simulink library "Enrg_conv_El_to_Mec_Bosch"  (R2016a)
settings: Solver=ode1  StartTime=0.0  StopTime=Inf  FixedStep=0.001  RelTol=1e-3
undefined symbols (not defined in the file): drvEmot_RefTqeMOT, FirstDrivenAxle_FirstDrivenAxleNoOfEmot, FMIKit, SecondDrivenAxle_SecondDrivenAxleNoOfEmot
libraries: Enrg_conv_El_to_Mec_Bosch x13, Electrical_converter x8
(part 4 of 5)

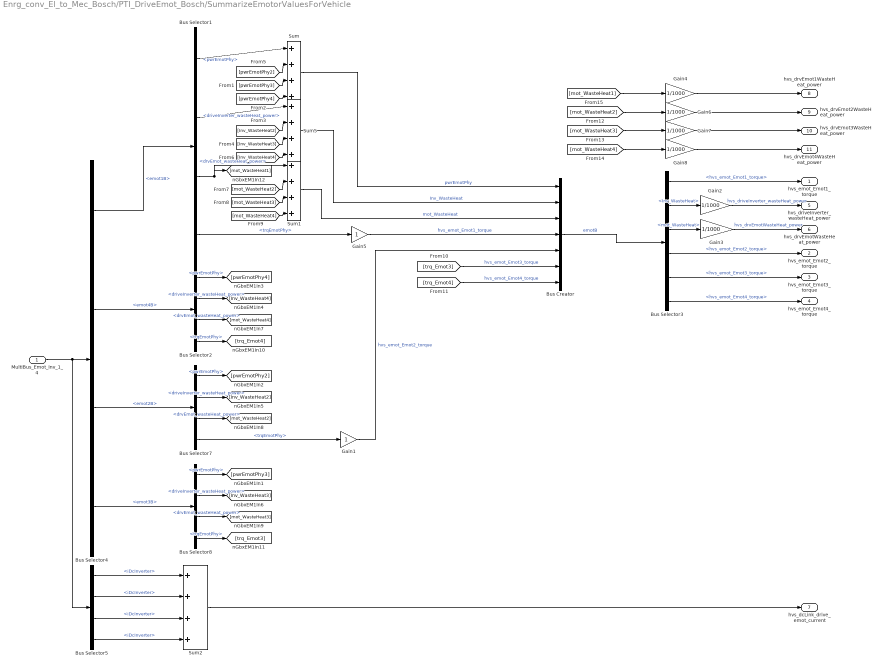
== system Enrg_conv_El_to_Mec_Bosch/PTI_DriveEmot_Bosch/SummarizeEmotorValuesForVehicle ==
  MultiBus_Emot_Inv_1_4 : Inport
  Bus Creator : BusCreator  Inputs=7
  Bus Selector{1..2,7..8} (4 alike) : BusSelector  OutputSignals=pwrEmotPhy,driveInverter_wasteHeat_power,drvEmot_wasteHeat_power,trqEmotPhy
  Bus Selector3 : BusSelector  OutputSignals=hvs_emot_Emot1_torque,Inv_WasteHeat,mot_WasteHeat,hvs_emot_Emot2_torque,hvs_emot_Emot3_torque,hvs_emot_Emot4_torque
  Bus Selector4 : BusSelector  OutputSignals=emot1_4B.emot1B,emot1_4B.emot4B,emot2_3B.emot2B,emot2_3B.emot3B
  Bus Selector5 : BusSelector  OutputSignals=emot1_4B.emot1B.iDcInverter,emot1_4B.emot4B.iDcInverter,emot2_3B.emot2B.iDcInverter,emot2_3B.emot3B.iDcInverter
  Gain1 : Gain
  Gain{2..4,6..8} (6 alike) : Gain  Gain=1/1000
  Gain5 : Gain
  Sum : Sum  Inputs=|++++
  Sum1 : Sum  Inputs=|++++
  Sum2 : Sum  Inputs=++++
  Sum5 : Sum  Inputs=|++++
  hvs_emot_Emot1_torque : Outport
  hvs_emot_Emot2_torque : Outport  Port=2
  hvs_emot_Emot3_torque : Outport  Port=3
  hvs_emot_Emot4_torque : Outport  Port=4
  hvs_driveInverter_wasteHeat_power : Outport  Port=5
  hvs_drvEmotWasteHeat_power : Outport  Port=6
  hvs_dcLink_drive_emot_current : Outport  Port=7
  hvs_drvEmot1WasteHeat_power : Outport  Port=8
  hvs_drvEmot2WasteHeat_power : Outport  Port=9
  hvs_drvEmot3WasteHeat_power : Outport  Port=10
  hvs_drvEmot4WasteHeat_power : Outport  Port=11
  wires:
  Gain5/1 -> Bus Creator/4  "hvs_emot_Emot1_torque"
  Sum1/1 -> Bus Creator/3  "mot_WasteHeat"
  Sum5/1 -> Bus Creator/2  "Inv_WasteHeat"
  Sum/1 -> Bus Creator/1  "pwrEmotPhy"
  Bus Selector1/4 -> Gain5/1  "<trqEmotPhy>"
  Bus Selector2/3 -> [mot_WasteHeat4]  "<drvEmot_wasteHeat_power>"
  Bus Selector1/3 -> [mot_WasteHeat1], Sum1/1  "<drvEmot_wasteHeat_power>"
  Bus Selector2/2 -> [Inv_WasteHeat4]  "<driveInverter_wasteHeat_power>"
  Bus Selector1/2 -> Sum5/1  "<driveInverter_wasteHeat_power>"
  Bus Selector1/1 -> Sum/1  "<pwrEmotPhy>"
  Bus Selector4/2 -> Bus Selector2/1  "<emot4B>"
  Bus Selector4/1 -> Bus Selector1/1  "<emot1B>"
  MultiBus_Emot_Inv_1_4/1 -> Bus Selector5/1, Bus Selector4/1
  Bus Creator/1 -> Bus Selector3/1  "emotB"
  Sum2/1 -> hvs_dcLink_drive_emot_current/1
  Bus Selector3/2 -> Gain2/1  "<Inv_WasteHeat>"
  Gain2/1 -> hvs_driveInverter_wasteHeat_power/1  "hvs_driveInverter_wasteHeat_power"
  Bus Selector3/3 -> Gain3/1  "<mot_WasteHeat>"
  Gain3/1 -> hvs_drvEmotWasteHeat_power/1  "hvs_drvEmotWasteHeat_power"
  Bus Selector4/4 -> Bus Selector8/1  "<emot3B>"
  Bus Selector4/3 -> Bus Selector7/1  "<emot2B>"
  Bus Selector7/1 -> [pwrEmotPhy2]  "<pwrEmotPhy>"
  Bus Selector8/1 -> [pwrEmotPhy3]  "<pwrEmotPhy>"
  Bus Selector2/1 -> [pwrEmotPhy4]  "<pwrEmotPhy>"
  [pwrEmotPhy2] -> Sum/2
  [pwrEmotPhy3] -> Sum/3
  [pwrEmotPhy4] -> Sum/4
  [Inv_WasteHeat2] -> Sum5/2
  [Inv_WasteHeat3] -> Sum5/3
  [Inv_WasteHeat4] -> Sum5/4
  Bus Selector7/2 -> [Inv_WasteHeat2]  "<driveInverter_wasteHeat_power>"
  Bus Selector8/2 -> [Inv_WasteHeat3]  "<driveInverter_wasteHeat_power>"
  Bus Selector7/3 -> [mot_WasteHeat2]  "<drvEmot_wasteHeat_power>"
  Bus Selector8/3 -> [mot_WasteHeat3]  "<drvEmot_wasteHeat_power>"
  [mot_WasteHeat2] -> Sum1/2
  [mot_WasteHeat3] -> Sum1/3
  [mot_WasteHeat4] -> Sum1/4
  Bus Selector7/4 -> Gain1/1  "<trqEmotPhy>"
  Bus Selector8/4 -> [trq_Emot3]  "<trqEmotPhy>"
  Gain1/1 -> Bus Creator/5  "hvs_emot_Emot2_torque"
  Bus Selector2/4 -> [trq_Emot4]  "<trqEmotPhy>"
  [trq_Emot3] -> Bus Creator/6  "hvs_emot_Emot3_torque"
  [trq_Emot4] -> Bus Creator/7  "hvs_emot_Emot4_torque"
  Bus Selector3/1 -> hvs_emot_Emot1_torque/1  "<hvs_emot_Emot1_torque>"
  Bus Selector3/4 -> hvs_emot_Emot2_torque/1  "<hvs_emot_Emot2_torque>"
  Bus Selector3/5 -> hvs_emot_Emot3_torque/1  "<hvs_emot_Emot3_torque>"
  Bus Selector3/6 -> hvs_emot_Emot4_torque/1  "<hvs_emot_Emot4_torque>"
  [mot_WasteHeat1] -> Gain4/1
  [mot_WasteHeat2] -> Gain6/1
  [mot_WasteHeat3] -> Gain7/1
  [mot_WasteHeat4] -> Gain8/1
  Gain4/1 -> hvs_drvEmot1WasteHeat_power/1
  Gain6/1 -> hvs_drvEmot2WasteHeat_power/1
  Gain7/1 -> hvs_drvEmot3WasteHeat_power/1
  Gain8/1 -> hvs_drvEmot4WasteHeat_power/1
  Bus Selector5/1 -> Sum2/1  "<iDcInverter>"
  Bus Selector5/3 -> Sum2/3  "<iDcInverter>"
  Bus Selector5/4 -> Sum2/4  "<iDcInverter>"
  Bus Selector5/2 -> Sum2/2  "<iDcInverter>"

== system Enrg_conv_El_to_Mec_Bosch/PTI_DriveEmot_Bosch_10ms/AWR1_4 ==
  EMD1_CMD_Commamd : Inport
  EMD1_CMD_MotorControlMode : Inport  Port=2
  EMD1_CMD_SpeedRefLim : Inport  Port=3
  EMD1_CMD_TorqueRefLim : Inport  Port=4
  HVFreigabeHW_SiRelay_D : Inport  Port=5
  vltZkBmsPhy : Inport  Port=6
  trqEmot1Phy : Inport  Port=7
  trqEmot4Phy : Inport  Port=8
  pwEmot1Phy : Inport  Port=9
  pwEmot4Phy : Inport  Port=10
  trqEmot1Max : Inport  Port=11
  trqEmot4Max : Inport  Port=12
  hvs_emot_Emot1_angVel : Inport  Port=13
  EMD4_CMD_Commamd : Inport  Port=14
  EMD4_CMD_MotorControlMode : Inport  Port=15
  EMD4_CMD_SpeedRefLim : Inport  Port=16
  EMD4_CMD_TorqueRefLim : Inport  Port=17
  HVFreigabeHW4_SiRelay_D : Inport  Port=18
  EDCU_Dig_SafetyCutOffDG1 : Inport  Port=19
  Emot1_Selection : Inport  Port=20
  Emot4_Selection : Inport  Port=21
  hvs_emot_Emot4_angVel : Inport  Port=22
  Bus Creator3 : BusCreator  Inputs=11
  Bus Creator4 : BusCreator  Inputs=2
  Bus Creator5 : BusCreator  Inputs=11
  Gain : Gain
  Gain1 : Gain
  Switch1 : Switch  Threshold=0.5
  Switch2 : Switch  Threshold=0.5
  ZeroWhenNotReady1 : Subsystem  TreatAsAtomicUnit=on
  ZeroWhenNotReady2 : Subsystem  TreatAsAtomicUnit=on
  awr1 : Electrical_converter/awr  SystemSampleTime=-1
  awr4 : Electrical_converter/awr  SystemSampleTime=-1
  awr1_4B : Outport
  wires:
  Emot1_Selection/1 -> awr1/Enable
  Emot4_Selection/1 -> awr4/Enable
  [EDCU_Dig_SafetyCutOffDG1] -> awr4/11
  EDCU_Dig_SafetyCutOffDG1/1 -> awr1/11, [EDCU_Dig_SafetyCutOffDG1]
  [vltZkBmsPhy] -> awr4/6
  EMD1_CMD_Commamd/1 -> awr1/1
  Bus Creator5/1 -> Switch2/1
  awr1/12 -> Switch2/2
  awr1/2 -> Bus Creator5/2
  awr1/3 -> Bus Creator5/3
  awr1/1 -> Gain/1
  awr1/4 -> Bus Creator5/4
  awr1/5 -> Bus Creator5/5
  awr1/8 -> Bus Creator5/8
  awr1/11 -> Bus Creator5/11
  awr1/10 -> Bus Creator5/10
  awr1/6 -> Bus Creator5/6
  awr1/7 -> Bus Creator5/7
  awr1/9 -> Bus Creator5/9
  awr4/12 -> Switch1/2
  Switch2/1 -> Bus Creator4/1  "awr1B"
  ZeroWhenNotReady1/1(Out1) -> Switch2/3
  awr4/4 -> Bus Creator3/4
  awr4/1 -> Gain1/1
  awr4/6 -> Bus Creator3/6
  awr4/7 -> Bus Creator3/7
  awr4/8 -> Bus Creator3/8
  awr4/9 -> Bus Creator3/9
  awr4/5 -> Bus Creator3/5
  awr4/11 -> Bus Creator3/11
  awr4/10 -> Bus Creator3/10
  awr4/3 -> Bus Creator3/3
  awr4/2 -> Bus Creator3/2
  Switch1/1 -> Bus Creator4/2  "awr4B"
  ZeroWhenNotReady2/1(Out1) -> Switch1/3
  Bus Creator3/1 -> Switch1/1  "awr4B"
  trqEmot1Max/1 -> awr1/9
  pwEmot1Phy/1 -> awr1/8
  trqEmot1Phy/1 -> awr1/7
  trqEmot4Max/1 -> awr4/9
  pwEmot4Phy/1 -> awr4/8
  trqEmot4Phy/1 -> awr4/7
  Bus Creator4/1 -> awr1_4B/1  "awr1_4B"
  EMD4_CMD_TorqueRefLim/1 -> awr4/4
  EMD4_CMD_Commamd/1 -> awr4/1
  EMD4_CMD_SpeedRefLim/1 -> awr4/3
  HVFreigabeHW4_SiRelay_D/1 -> awr4/5
  HVFreigabeHW_SiRelay_D/1 -> awr1/5
  EMD1_CMD_TorqueRefLim/1 -> awr1/4
  EMD1_CMD_SpeedRefLim/1 -> awr1/3
  Gain/1 -> Bus Creator5/1  "EMD1_ACT_DcLinkVoltage"
  Gain1/1 -> Bus Creator3/1  "EMD4_ACT_DcLinkVoltage"
  hvs_emot_Emot4_angVel/1 -> awr4/10
  EMD4_CMD_MotorControlMode/1 -> awr4/2
  EMD1_CMD_MotorControlMode/1 -> awr1/2
  vltZkBmsPhy/1 -> awr1/6, [vltZkBmsPhy]
  hvs_emot_Emot1_angVel/1 -> awr1/10

== system Enrg_conv_El_to_Mec_Bosch/PTI_DriveEmot_Bosch_10ms/AWR2_3 ==
  EMD2_CMD_Commamd : Inport
  EMD2_CMD_MotorControlMode : Inport  Port=2
  EMD2_CMD_SpeedRefLim : Inport  Port=3
  EMD2_CMD_TorqueRefLim : Inport  Port=4
  HVFreigabeHW2_SiRelay_D : Inport  Port=5
  vltZkBmsPhy : Inport  Port=6
  trqEmot2Phy : Inport  Port=7
  trqEmot3Phy : Inport  Port=8
  pwEmot2Phy : Inport  Port=9
  pwEmot3Phy : Inport  Port=10
  trqEmot2Max : Inport  Port=11
  trqEmot3Max : Inport  Port=12
  hvs_emot_Emot2_angVel : Inport  Port=13
  EMD3_CMD_Commamd : Inport  Port=14
  EMD3_CMD_MotorControlMode : Inport  Port=15
  EMD3_CMD_SpeedRefLim : Inport  Port=16
  EMD3_CMD_TorqueRefLim : Inport  Port=17
  HVFreigabeHW3_SiRelay_D : Inport  Port=18
  EDCU_Dig_SafetyCutOffDG1 : Inport  Port=19
  Emot2_Selection : Inport  Port=20
  Emot3_Selection : Inport  Port=21
  hvs_emot_Emot3_angVel : Inport  Port=22
  Bus Creator3 : BusCreator  Inputs=11
  Bus Creator4 : BusCreator  Inputs=2
  Bus Creator5 : BusCreator  Inputs=11
  Gain : Gain
  Gain1 : Gain
  Switch1 : Switch  Threshold=0.5
  Switch2 : Switch  Threshold=0.5
  ZeroWhenNotReady1 : Subsystem  TreatAsAtomicUnit=on
  ZeroWhenNotReady2 : Subsystem  TreatAsAtomicUnit=on
  awr2 : Electrical_converter/awr  SystemSampleTime=-1
  awr3 : Electrical_converter/awr  SystemSampleTime=-1
  awr2_3B : Outport
  wires:
  Emot3_Selection/1 -> awr3/Enable
  Emot2_Selection/1 -> awr2/Enable
  [EDCU_Dig_SafetyCutOffDG1] -> awr3/11
  EDCU_Dig_SafetyCutOffDG1/1 -> awr2/11, [EDCU_Dig_SafetyCutOffDG1]
  hvs_emot_Emot2_angVel/1 -> awr2/10
  vltZkBmsPhy/1 -> [vltZkBmsPhy], awr2/6
  EMD2_CMD_MotorControlMode/1 -> awr2/2
  EMD3_CMD_MotorControlMode/1 -> awr3/2
  hvs_emot_Emot3_angVel/1 -> awr3/10
  Gain1/1 -> Bus Creator3/1  "EMD3_ACT_DcLinkVoltage"
  Gain/1 -> Bus Creator5/1  "EMD2_ACT_DcLinkVoltage"
  EMD2_CMD_SpeedRefLim/1 -> awr2/3
  EMD2_CMD_TorqueRefLim/1 -> awr2/4
  HVFreigabeHW2_SiRelay_D/1 -> awr2/5
  HVFreigabeHW3_SiRelay_D/1 -> awr3/5
  EMD3_CMD_SpeedRefLim/1 -> awr3/3
  EMD3_CMD_Commamd/1 -> awr3/1
  EMD3_CMD_TorqueRefLim/1 -> awr3/4
  Bus Creator4/1 -> awr2_3B/1  "awr2_3B"
  trqEmot3Phy/1 -> awr3/7
  pwEmot3Phy/1 -> awr3/8
  trqEmot3Max/1 -> awr3/9
  trqEmot2Phy/1 -> awr2/7
  pwEmot2Phy/1 -> awr2/8
  trqEmot2Max/1 -> awr2/9
  Bus Creator3/1 -> Switch1/1  "awr3B"
  ZeroWhenNotReady2/1(Out1) -> Switch1/3
  Switch1/1 -> Bus Creator4/2  "awr3B"
  awr3/2 -> Bus Creator3/2
  awr3/3 -> Bus Creator3/3
  awr3/10 -> Bus Creator3/10
  awr3/11 -> Bus Creator3/11
  awr3/5 -> Bus Creator3/5
  awr3/9 -> Bus Creator3/9
  awr3/8 -> Bus Creator3/8
  awr3/7 -> Bus Creator3/7
  awr3/6 -> Bus Creator3/6
  awr3/1 -> Gain1/1
  awr3/4 -> Bus Creator3/4
  ZeroWhenNotReady1/1(Out1) -> Switch2/3
  Switch2/1 -> Bus Creator4/1  "awr2B"
  awr3/12 -> Switch1/2
  awr2/9 -> Bus Creator5/9
  awr2/7 -> Bus Creator5/7
  awr2/6 -> Bus Creator5/6
  awr2/10 -> Bus Creator5/10
  awr2/11 -> Bus Creator5/11
  awr2/8 -> Bus Creator5/8
  awr2/5 -> Bus Creator5/5
  awr2/4 -> Bus Creator5/4
  awr2/1 -> Gain/1
  awr2/3 -> Bus Creator5/3
  awr2/2 -> Bus Creator5/2
  awr2/12 -> Switch2/2
  Bus Creator5/1 -> Switch2/1
  EMD2_CMD_Commamd/1 -> awr2/1
  [vltZkBmsPhy] -> awr3/6

== system Enrg_conv_El_to_Mec_Bosch/PTI_DriveEmot_Bosch_10ms/EMD1_CMD_Command ==
  EMD1_CMD_ClearErrors : Inport
  EMD1_CMD_MotorControlMode : Inport  Port=2
  Compare To Constant : Subsystem  mask(Compare To Constant){relop===, const=1, OutDataTypeStr=boolean, ZeroCross=on}
      mask prompts: relop "Simulink:masks:Operator_MP"; const "Simulink:masks:ConstantValue_MP"; OutDataTypeStr "Simulink:masks:OutputDataType_MP"; ZeroCross "Simulink:masks:EnableZerocrossingDetection_MP"
      mask help: Simulink:masks:CompareToConstant_MD
      mask init: same as Enrg_conv_El_to_Mec_Bosch/PTI_DriveEmot_Bosch/EMD1_CMD_Command/Compare To Constant
      mask TypeOptions relop: == | ~= | < | <= | >= | >
      mask TypeOptions OutDataTypeStr: Simulink:masks:uint8 | Simulink:masks:boolean
      mask Callback ZeroCross: sl('zeroCrossEnable', gcbh);
      mask Display: disp(str)
  Compare To Constant1 : Subsystem  mask(Compare To Constant){relop===, const=1, OutDataTypeStr=boolean, ZeroCross=on}
      mask prompts: relop "Simulink:masks:Operator_MP"; const "Simulink:masks:ConstantValue_MP"; OutDataTypeStr "Simulink:masks:OutputDataType_MP"; ZeroCross "Simulink:masks:EnableZerocrossingDetection_MP"
      mask help: Simulink:masks:CompareToConstant_MD
      mask init: same as Enrg_conv_El_to_Mec_Bosch/PTI_DriveEmot_Bosch/EMD1_CMD_Command/Compare To Constant
      mask TypeOptions relop: == | ~= | < | <= | >= | >
      mask TypeOptions OutDataTypeStr: Simulink:masks:uint8 | Simulink:masks:boolean
      mask Callback ZeroCross: sl('zeroCrossEnable', gcbh);
      mask Display: disp(str)
  Constant : Constant  Value=4
  Constant3 : Constant
  Constant4 : Constant  Value=0
  Switch : Switch  Threshold=0.5
  Switch1 : Switch  Threshold=0.5
  Out_EMD1_CMD_Command : Outport
  wires:
  EMD1_CMD_MotorControlMode/1 -> Compare To Constant/1(u)
  EMD1_CMD_ClearErrors/1 -> Compare To Constant1/1(u)
  Compare To Constant1/1(y) -> Switch/2
  Switch1/1 -> Switch/3
  Constant/1 -> Switch/1
  Constant3/1 -> Switch1/1
  Constant4/1 -> Switch1/3
  Switch/1 -> Out_EMD1_CMD_Command/1
  Compare To Constant/1(y) -> Switch1/2

== system Enrg_conv_El_to_Mec_Bosch/PTI_DriveEmot_Bosch_10ms/EMD1_CMD_Command1 ==
  EMD1_CMD_ClearErrors : Inport
  EMD1_CMD_MotorControlMode : Inport  Port=2
  Compare To Constant : Subsystem  mask(Compare To Constant){relop===, const=1, OutDataTypeStr=boolean, ZeroCross=on}
      mask prompts: relop "Simulink:masks:Operator_MP"; const "Simulink:masks:ConstantValue_MP"; OutDataTypeStr "Simulink:masks:OutputDataType_MP"; ZeroCross "Simulink:masks:EnableZerocrossingDetection_MP"
      mask help: Simulink:masks:CompareToConstant_MD
      mask init: same as Enrg_conv_El_to_Mec_Bosch/PTI_DriveEmot_Bosch/EMD1_CMD_Command/Compare To Constant
      mask TypeOptions relop: == | ~= | < | <= | >= | >
      mask TypeOptions OutDataTypeStr: Simulink:masks:uint8 | Simulink:masks:boolean
      mask Callback ZeroCross: sl('zeroCrossEnable', gcbh);
      mask Display: disp(str)
  Compare To Constant1 : Subsystem  mask(Compare To Constant){relop===, const=1, OutDataTypeStr=boolean, ZeroCross=on}
      mask prompts: relop "Simulink:masks:Operator_MP"; const "Simulink:masks:ConstantValue_MP"; OutDataTypeStr "Simulink:masks:OutputDataType_MP"; ZeroCross "Simulink:masks:EnableZerocrossingDetection_MP"
      mask help: Simulink:masks:CompareToConstant_MD
      mask init: same as Enrg_conv_El_to_Mec_Bosch/PTI_DriveEmot_Bosch/EMD1_CMD_Command/Compare To Constant
      mask TypeOptions relop: == | ~= | < | <= | >= | >
      mask TypeOptions OutDataTypeStr: Simulink:masks:uint8 | Simulink:masks:boolean
      mask Callback ZeroCross: sl('zeroCrossEnable', gcbh);
      mask Display: disp(str)
  Constant : Constant  Value=4
  Constant3 : Constant
  Constant4 : Constant  Value=0
  Switch : Switch  Threshold=0.5
  Switch1 : Switch  Threshold=0.5
  Out_EMD1_CMD_Command : Outport
  wires:
  EMD1_CMD_MotorControlMode/1 -> Compare To Constant/1(u)
  EMD1_CMD_ClearErrors/1 -> Compare To Constant1/1(u)
  Compare To Constant1/1(y) -> Switch/2
  Switch1/1 -> Switch/3
  Constant/1 -> Switch/1
  Constant3/1 -> Switch1/1
  Constant4/1 -> Switch1/3
  Switch/1 -> Out_EMD1_CMD_Command/1
  Compare To Constant/1(y) -> Switch1/2

== system Enrg_conv_El_to_Mec_Bosch/PTI_DriveEmot_Bosch_10ms/EMD1_CMD_Command2 ==
  EMD1_CMD_ClearErrors : Inport
  EMD1_CMD_MotorControlMode : Inport  Port=2
  Compare To Constant : Subsystem  mask(Compare To Constant){relop===, const=1, OutDataTypeStr=boolean, ZeroCross=on}
      mask prompts: relop "Simulink:masks:Operator_MP"; const "Simulink:masks:ConstantValue_MP"; OutDataTypeStr "Simulink:masks:OutputDataType_MP"; ZeroCross "Simulink:masks:EnableZerocrossingDetection_MP"
      mask help: Simulink:masks:CompareToConstant_MD
      mask init: same as Enrg_conv_El_to_Mec_Bosch/PTI_DriveEmot_Bosch/EMD1_CMD_Command/Compare To Constant
      mask TypeOptions relop: == | ~= | < | <= | >= | >
      mask TypeOptions OutDataTypeStr: Simulink:masks:uint8 | Simulink:masks:boolean
      mask Callback ZeroCross: sl('zeroCrossEnable', gcbh);
      mask Display: disp(str)
  Compare To Constant1 : Subsystem  mask(Compare To Constant){relop===, const=1, OutDataTypeStr=boolean, ZeroCross=on}
      mask prompts: relop "Simulink:masks:Operator_MP"; const "Simulink:masks:ConstantValue_MP"; OutDataTypeStr "Simulink:masks:OutputDataType_MP"; ZeroCross "Simulink:masks:EnableZerocrossingDetection_MP"
      mask help: Simulink:masks:CompareToConstant_MD
      mask init: same as Enrg_conv_El_to_Mec_Bosch/PTI_DriveEmot_Bosch/EMD1_CMD_Command/Compare To Constant
      mask TypeOptions relop: == | ~= | < | <= | >= | >
      mask TypeOptions OutDataTypeStr: Simulink:masks:uint8 | Simulink:masks:boolean
      mask Callback ZeroCross: sl('zeroCrossEnable', gcbh);
      mask Display: disp(str)
  Constant : Constant  Value=4
  Constant3 : Constant
  Constant4 : Constant  Value=0
  Switch : Switch  Threshold=0.5
  Switch1 : Switch  Threshold=0.5
  Out_EMD1_CMD_Command : Outport
  wires:
  EMD1_CMD_MotorControlMode/1 -> Compare To Constant/1(u)
  EMD1_CMD_ClearErrors/1 -> Compare To Constant1/1(u)
  Compare To Constant1/1(y) -> Switch/2
  Switch1/1 -> Switch/3
  Constant/1 -> Switch/1
  Constant3/1 -> Switch1/1
  Constant4/1 -> Switch1/3
  Switch/1 -> Out_EMD1_CMD_Command/1
  Compare To Constant/1(y) -> Switch1/2

== system Enrg_conv_El_to_Mec_Bosch/PTI_DriveEmot_Bosch_10ms/EMD1_CMD_Command3 ==
  EMD1_CMD_ClearErrors : Inport
  EMD1_CMD_MotorControlMode : Inport  Port=2
  Compare To Constant : Subsystem  mask(Compare To Constant){relop===, const=1, OutDataTypeStr=boolean, ZeroCross=on}
      mask prompts: relop "Simulink:masks:Operator_MP"; const "Simulink:masks:ConstantValue_MP"; OutDataTypeStr "Simulink:masks:OutputDataType_MP"; ZeroCross "Simulink:masks:EnableZerocrossingDetection_MP"
      mask help: Simulink:masks:CompareToConstant_MD
      mask init: same as Enrg_conv_El_to_Mec_Bosch/PTI_DriveEmot_Bosch/EMD1_CMD_Command/Compare To Constant
      mask TypeOptions relop: == | ~= | < | <= | >= | >
      mask TypeOptions OutDataTypeStr: Simulink:masks:uint8 | Simulink:masks:boolean
      mask Callback ZeroCross: sl('zeroCrossEnable', gcbh);
      mask Display: disp(str)
  Compare To Constant1 : Subsystem  mask(Compare To Constant){relop===, const=1, OutDataTypeStr=boolean, ZeroCross=on}
      mask prompts: relop "Simulink:masks:Operator_MP"; const "Simulink:masks:ConstantValue_MP"; OutDataTypeStr "Simulink:masks:OutputDataType_MP"; ZeroCross "Simulink:masks:EnableZerocrossingDetection_MP"
      mask help: Simulink:masks:CompareToConstant_MD
      mask init: same as Enrg_conv_El_to_Mec_Bosch/PTI_DriveEmot_Bosch/EMD1_CMD_Command/Compare To Constant
      mask TypeOptions relop: == | ~= | < | <= | >= | >
      mask TypeOptions OutDataTypeStr: Simulink:masks:uint8 | Simulink:masks:boolean
      mask Callback ZeroCross: sl('zeroCrossEnable', gcbh);
      mask Display: disp(str)
  Constant : Constant  Value=4
  Constant3 : Constant
  Constant4 : Constant  Value=0
  Switch : Switch  Threshold=0.5
  Switch1 : Switch  Threshold=0.5
  Out_EMD1_CMD_Command : Outport
  wires:
  EMD1_CMD_MotorControlMode/1 -> Compare To Constant/1(u)
  EMD1_CMD_ClearErrors/1 -> Compare To Constant1/1(u)
  Compare To Constant1/1(y) -> Switch/2
  Switch1/1 -> Switch/3
  Constant/1 -> Switch/1
  Constant3/1 -> Switch1/1
  Constant4/1 -> Switch1/3
  Switch/1 -> Out_EMD1_CMD_Command/1
  Compare To Constant/1(y) -> Switch1/2

== system Enrg_conv_El_to_Mec_Bosch/PTI_DriveEmot_Bosch_10ms/Emot1_4 ==
  emot_Emot1_angVel : Inport
  voltBatHV1 : Inport  Port=2
  trqEmotDesPhy1 : Inport  Port=3
  voltBatHV4 : Inport  Port=4
  trqEmotDesPhy4 : Inport  Port=5
  drvEmot1_Oil_Temperature : Inport  Port=6
  drvEmot1_Coolant_Temperature : Inport  Port=7
  drvEmot_Ambient_Temperature : Inport  Port=8
  inv_coolant_temperature : Inport  Port=9
  inv1_switching_freq : Inport  Port=10
  inv4_switching_freq : Inport  Port=11
  emot_Emot4_angVel : Inport  Port=12
  drvEmot4_Oil_Temperature : Inport  Port=13
  drvEmot4_Coolant_Temperature : Inport  Port=14
  Emot1_Selection : Inport  Port=15
  Emot4_Selection : Inport  Port=16
  drvEmot1CoolantFlow_vdot : Inport  Port=17
  drvEmot1OilFlow_vdot : Inport  Port=18
  driveInverterCoolantFlow_vdot : Inport  Port=19
  drvEmot4CoolantFlow_vdot : Inport  Port=20
  drvEmot4OilFlow_vdot : Inport  Port=21
  Bus Creator1 : BusCreator  Inputs=17
  Bus Creator2 : BusCreator  Inputs=17
  Bus Creator3 : BusCreator  Inputs=2
  e-Motor 1 Bosch 10ms : Enrg_conv_El_to_Mec_Bosch/e-Motor Bosch 10ms  SystemSampleTime=-1
  e-Motor 4 Bosch 10ms : Enrg_conv_El_to_Mec_Bosch/e-Motor Bosch 10ms  SystemSampleTime=-1
  emot1_4B : Outport
  wires:
  inv4_switching_freq/1 -> e-Motor 4 Bosch 10ms/8
  drvEmot4_Coolant_Temperature/1 -> e-Motor 4 Bosch 10ms/5
  inv1_switching_freq/1 -> e-Motor 1 Bosch 10ms/8
  drvEmot_Ambient_Temperature/1 -> e-Motor 1 Bosch 10ms/6, e-Motor 4 Bosch 10ms/6
  drvEmot1_Coolant_Temperature/1 -> e-Motor 1 Bosch 10ms/5
  drvEmot4_Oil_Temperature/1 -> e-Motor 4 Bosch 10ms/4
  Emot1_Selection/1 -> e-Motor 1 Bosch 10ms/Enable
  Emot4_Selection/1 -> e-Motor 4 Bosch 10ms/Enable
  Bus Creator3/1 -> emot1_4B/1  "emot1_4B"
  trqEmotDesPhy4/1 -> e-Motor 4 Bosch 10ms/3
  voltBatHV4/1 -> e-Motor 4 Bosch 10ms/2
  emot_Emot4_angVel/1 -> e-Motor 4 Bosch 10ms/1
  voltBatHV1/1 -> e-Motor 1 Bosch 10ms/2
  trqEmotDesPhy1/1 -> e-Motor 1 Bosch 10ms/3
  emot_Emot1_angVel/1 -> e-Motor 1 Bosch 10ms/1
  inv_coolant_temperature/1 -> e-Motor 4 Bosch 10ms/7, e-Motor 1 Bosch 10ms/7
  drvEmot1_Oil_Temperature/1 -> e-Motor 1 Bosch 10ms/4
  drvEmot1CoolantFlow_vdot/1 -> e-Motor 1 Bosch 10ms/9
  drvEmot1OilFlow_vdot/1 -> e-Motor 1 Bosch 10ms/10
  driveInverterCoolantFlow_vdot/1 -> e-Motor 4 Bosch 10ms/11, e-Motor 1 Bosch 10ms/11
  drvEmot4CoolantFlow_vdot/1 -> e-Motor 4 Bosch 10ms/9
  drvEmot4OilFlow_vdot/1 -> e-Motor 4 Bosch 10ms/10
  e-Motor 1 Bosch 10ms/1 -> Bus Creator1/1  "pwrEmotPhy"
  Bus Creator1/1 -> Bus Creator3/1  "emot1B"
  e-Motor 1 Bosch 10ms/13 -> Bus Creator1/13  "iStator"
  e-Motor 1 Bosch 10ms/9 -> Bus Creator1/9  "driveInverter_wasteHeat_power"
  e-Motor 1 Bosch 10ms/10 -> Bus Creator1/10  "driveInverter_Temperatures"
  e-Motor 1 Bosch 10ms/8 -> Bus Creator1/8  "drvEmot_T_Stator"
  e-Motor 1 Bosch 10ms/7 -> Bus Creator1/7  "drvEmot_wasteHeat_power"
  e-Motor 1 Bosch 10ms/6 -> Bus Creator1/6  "trqEmotMax"
  e-Motor 1 Bosch 10ms/3 -> Bus Creator1/3  "Inv_Ploss"
  e-Motor 1 Bosch 10ms/5 -> Bus Creator1/5  "trqEmotPhy"
  e-Motor 1 Bosch 10ms/4 -> Bus Creator1/4  "mot_Ploss"
  e-Motor 1 Bosch 10ms/11 -> Bus Creator1/11  "drvEmot_T_Rotor"
  e-Motor 1 Bosch 10ms/12 -> Bus Creator1/12  "uStator"
  e-Motor 1 Bosch 10ms/2 -> Bus Creator1/2  "iDcInverter"
  e-Motor 1 Bosch 10ms/14 -> Bus Creator1/14  "modIdx"
  e-Motor 1 Bosch 10ms/15 -> Bus Creator1/15  "cosPhi"
  e-Motor 1 Bosch 10ms/16 -> Bus Creator1/16  "wasteHeat_coolant"
  e-Motor 1 Bosch 10ms/17 -> Bus Creator1/17  "wasteHeat_oil"
  Bus Creator2/1 -> Bus Creator3/2  "emot4B"
  e-Motor 4 Bosch 10ms/1 -> Bus Creator2/1  "pwrEmotPhy"
  e-Motor 4 Bosch 10ms/13 -> Bus Creator2/13  "iStator"
  e-Motor 4 Bosch 10ms/9 -> Bus Creator2/9  "driveInverter_wasteHeat_power"
  e-Motor 4 Bosch 10ms/10 -> Bus Creator2/10  "driveInverter_Temperatures"
  e-Motor 4 Bosch 10ms/8 -> Bus Creator2/8  "drvEmot_T_Stator"
  e-Motor 4 Bosch 10ms/7 -> Bus Creator2/7  "drvEmot_wasteHeat_power"
  e-Motor 4 Bosch 10ms/6 -> Bus Creator2/6  "trqEmotMax"
  e-Motor 4 Bosch 10ms/3 -> Bus Creator2/3  "Inv_Ploss"
  e-Motor 4 Bosch 10ms/5 -> Bus Creator2/5  "trqEmotPhy"
  e-Motor 4 Bosch 10ms/4 -> Bus Creator2/4  "mot_Ploss"
  e-Motor 4 Bosch 10ms/11 -> Bus Creator2/11  "drvEmot_T_Rotor"
  e-Motor 4 Bosch 10ms/12 -> Bus Creator2/12  "uStator"
  e-Motor 4 Bosch 10ms/2 -> Bus Creator2/2  "iDcInverter"
  e-Motor 4 Bosch 10ms/14 -> Bus Creator2/14  "modIdx"
  e-Motor 4 Bosch 10ms/15 -> Bus Creator2/15  "cosPhi"
  e-Motor 4 Bosch 10ms/16 -> Bus Creator2/16  "wasteHeat_coolant"
  e-Motor 4 Bosch 10ms/17 -> Bus Creator2/17  "wasteHeat_oil"

== system Enrg_conv_El_to_Mec_Bosch/PTI_DriveEmot_Bosch_10ms/Emot2_3 ==
  emot_Emot2_angVel : Inport
  voltBatHV2 : Inport  Port=2
  trqEmotDesPhy2 : Inport  Port=3
  voltBatHV3 : Inport  Port=4
  trqEmotDesPhy3 : Inport  Port=5
  drvEmot2_Oil_Temperature : Inport  Port=6
  drvEmot2_Coolant_Temperature : Inport  Port=7
  drvEmot_Ambient_Temperature : Inport  Port=8
  inv_coolant_temperature : Inport  Port=9
  inv2_switching_freq : Inport  Port=10
  inv3_switching_freq : Inport  Port=11
  emot_Emot3_angVel : Inport  Port=12
  drvEmot3_Oil_Temperature : Inport  Port=13
  drvEmot3_Coolant_Temperature : Inport  Port=14
  Emot2_Selection : Inport  Port=15
  Emot3_Selection : Inport  Port=16
  drvEmot2CoolantFlow_vdot : Inport  Port=17
  drvEmot2OilFlow_vdot : Inport  Port=18
  driveInverterCoolantFlow_vdot : Inport  Port=19
  drvEmot3CoolantFlow_vdot : Inport  Port=20
  drvEmot3OilFlow_vdot : Inport  Port=21
  Bus Creator1 : BusCreator  Inputs=17
  Bus Creator2 : BusCreator  Inputs=17
  Bus Creator3 : BusCreator  Inputs=2
  e-Motor 2 Bosch 10ms : Enrg_conv_El_to_Mec_Bosch/e-Motor Bosch 10ms  SystemSampleTime=-1
  e-Motor 3 Bosch 10ms : Enrg_conv_El_to_Mec_Bosch/e-Motor Bosch 10ms  SystemSampleTime=-1
  emot2_3B : Outport
  wires:
  inv3_switching_freq/1 -> e-Motor 3 Bosch 10ms/8
  Emot3_Selection/1 -> e-Motor 3 Bosch 10ms/Enable
  drvEmot3_Coolant_Temperature/1 -> e-Motor 3 Bosch 10ms/5
  drvEmot3_Oil_Temperature/1 -> e-Motor 3 Bosch 10ms/4
  trqEmotDesPhy3/1 -> e-Motor 3 Bosch 10ms/3
  voltBatHV3/1 -> e-Motor 3 Bosch 10ms/2
  emot_Emot3_angVel/1 -> e-Motor 3 Bosch 10ms/1
  inv2_switching_freq/1 -> e-Motor 2 Bosch 10ms/8
  drvEmot_Ambient_Temperature/1 -> e-Motor 3 Bosch 10ms/6, e-Motor 2 Bosch 10ms/6
  drvEmot2_Coolant_Temperature/1 -> e-Motor 2 Bosch 10ms/5
  Emot2_Selection/1 -> e-Motor 2 Bosch 10ms/Enable
  voltBatHV2/1 -> e-Motor 2 Bosch 10ms/2
  trqEmotDesPhy2/1 -> e-Motor 2 Bosch 10ms/3
  emot_Emot2_angVel/1 -> e-Motor 2 Bosch 10ms/1
  inv_coolant_temperature/1 -> e-Motor 3 Bosch 10ms/7, e-Motor 2 Bosch 10ms/7
  drvEmot2_Oil_Temperature/1 -> e-Motor 2 Bosch 10ms/4
  Bus Creator3/1 -> emot2_3B/1  "emot2_3B"
  driveInverterCoolantFlow_vdot/1 -> e-Motor 3 Bosch 10ms/11, e-Motor 2 Bosch 10ms/11
  drvEmot2CoolantFlow_vdot/1 -> e-Motor 2 Bosch 10ms/9
  drvEmot2OilFlow_vdot/1 -> e-Motor 2 Bosch 10ms/10
  drvEmot3CoolantFlow_vdot/1 -> e-Motor 3 Bosch 10ms/9
  drvEmot3OilFlow_vdot/1 -> e-Motor 3 Bosch 10ms/10
  e-Motor 2 Bosch 10ms/1 -> Bus Creator1/1  "pwrEmotPhy"
  Bus Creator1/1 -> Bus Creator3/1  "emot2B"
  e-Motor 2 Bosch 10ms/13 -> Bus Creator1/13  "iStator"
  e-Motor 2 Bosch 10ms/9 -> Bus Creator1/9  "driveInverter_wasteHeat_power"
  e-Motor 2 Bosch 10ms/10 -> Bus Creator1/10  "driveInverter_Temperatures"
  e-Motor 2 Bosch 10ms/8 -> Bus Creator1/8  "drvEmot_T_Stator"
  e-Motor 2 Bosch 10ms/7 -> Bus Creator1/7  "drvEmot_wasteHeat_power"
  e-Motor 2 Bosch 10ms/6 -> Bus Creator1/6  "trqEmotMax"
  e-Motor 2 Bosch 10ms/3 -> Bus Creator1/3  "Inv_Ploss"
  e-Motor 2 Bosch 10ms/5 -> Bus Creator1/5  "trqEmotPhy"
  e-Motor 2 Bosch 10ms/4 -> Bus Creator1/4  "mot_Ploss"
  e-Motor 2 Bosch 10ms/11 -> Bus Creator1/11  "drvEmot_T_Rotor"
  e-Motor 2 Bosch 10ms/12 -> Bus Creator1/12  "uStator"
  e-Motor 2 Bosch 10ms/2 -> Bus Creator1/2  "iDcInverter"
  e-Motor 2 Bosch 10ms/14 -> Bus Creator1/14  "modIdx"
  e-Motor 2 Bosch 10ms/15 -> Bus Creator1/15  "cosPhi"
  e-Motor 2 Bosch 10ms/16 -> Bus Creator1/16  "wasteHeat_coolant"
  e-Motor 2 Bosch 10ms/17 -> Bus Creator1/17  "wasteHeat_oil"
  Bus Creator2/1 -> Bus Creator3/2  "emot3B"
  e-Motor 3 Bosch 10ms/1 -> Bus Creator2/1  "pwrEmotPhy"
  e-Motor 3 Bosch 10ms/13 -> Bus Creator2/13  "iStator"
  e-Motor 3 Bosch 10ms/9 -> Bus Creator2/9  "driveInverter_wasteHeat_power"
  e-Motor 3 Bosch 10ms/10 -> Bus Creator2/10  "driveInverter_Temperatures"
  e-Motor 3 Bosch 10ms/8 -> Bus Creator2/8  "drvEmot_T_Stator"
  e-Motor 3 Bosch 10ms/7 -> Bus Creator2/7  "drvEmot_wasteHeat_power"
  e-Motor 3 Bosch 10ms/6 -> Bus Creator2/6  "trqEmotMax"
  e-Motor 3 Bosch 10ms/3 -> Bus Creator2/3  "Inv_Ploss"
  e-Motor 3 Bosch 10ms/5 -> Bus Creator2/5  "trqEmotPhy"
  e-Motor 3 Bosch 10ms/4 -> Bus Creator2/4  "mot_Ploss"
  e-Motor 3 Bosch 10ms/11 -> Bus Creator2/11  "drvEmot_T_Rotor"
  e-Motor 3 Bosch 10ms/12 -> Bus Creator2/12  "uStator"
  e-Motor 3 Bosch 10ms/2 -> Bus Creator2/2  "iDcInverter"
  e-Motor 3 Bosch 10ms/14 -> Bus Creator2/14  "modIdx"
  e-Motor 3 Bosch 10ms/15 -> Bus Creator2/15  "cosPhi"
  e-Motor 3 Bosch 10ms/16 -> Bus Creator2/16  "wasteHeat_coolant"
  e-Motor 3 Bosch 10ms/17 -> Bus Creator2/17  "wasteHeat_oil"

== system Enrg_conv_El_to_Mec_Bosch/PTI_DriveEmot_Bosch_10ms/MotorSelection ==
  MidAxle : Constant  Value=FirstDrivenAxle_FirstDrivenAxleNoOfEmot
  RearAxle : Constant  Value=SecondDrivenAxle_SecondDrivenAxleNoOfEmot
  Truth Table : Truth Table  TreatAsAtomicUnit=on
  Emot1_Selection : Outport
  Emot2_Selection : Outport  Port=2
  Emot3_Selection : Outport  Port=3
  Emot4_Selection : Outport  Port=4
  wires:
  Truth Table/4(y4) -> Emot4_Selection/1
  Truth Table/3(y3) -> Emot3_Selection/1
  Truth Table/2(y2) -> Emot2_Selection/1
  Truth Table/1(y1) -> Emot1_Selection/1
  RearAxle/1 -> Truth Table/2(u2)
  MidAxle/1 -> Truth Table/1(u1)

== system Enrg_conv_El_to_Mec_Bosch/PTI_DriveEmot_Bosch/AWR 1 TX/Nm_to_percent ==
  Nm_Torque : Inport
  Reference_Torque : Inport  Port=2
  Constant : Constant  Value=100
  Divide1 : Product  Inputs=*/
  Product1 : Product  RndMeth=Zero
  Torque_Percentage : Outport
  wires:
  Nm_Torque/1 -> Divide1/1  "Nm_Torque"
  Product1/1 -> Torque_Percentage/1  "Torque_Percentage"
  Reference_Torque/1 -> Divide1/2  "Reference_Torque"
  Divide1/1 -> Product1/1
  Constant/1 -> Product1/2

== system Enrg_conv_El_to_Mec_Bosch/PTI_DriveEmot_Bosch/AWR 1 TX/Nm_to_percent1 ==
  Nm_Torque : Inport
  Reference_Torque : Inport  Port=2
  Constant : Constant  Value=100
  Divide1 : Product  Inputs=*/
  Product1 : Product  RndMeth=Zero
  Torque_Percentage : Outport
  wires:
  Constant/1 -> Product1/2
  Divide1/1 -> Product1/1
  Reference_Torque/1 -> Divide1/2  "Reference_Torque"
  Product1/1 -> Torque_Percentage/1  "Torque_Percentage"
  Nm_Torque/1 -> Divide1/1  "Nm_Torque"

== system Enrg_conv_El_to_Mec_Bosch/PTI_DriveEmot_Bosch/AWR 1 TX/Nm_to_percent2 ==
  Nm_Torque : Inport
  Reference_Torque : Inport  Port=2
  Constant : Constant  Value=100
  Divide1 : Product  Inputs=*/
  Product1 : Product  RndMeth=Zero
  Torque_Percentage : Outport
  wires:
  Nm_Torque/1 -> Divide1/1  "Nm_Torque"
  Product1/1 -> Torque_Percentage/1  "Torque_Percentage"
  Reference_Torque/1 -> Divide1/2  "Reference_Torque"
  Divide1/1 -> Product1/1
  Constant/1 -> Product1/2

== system Enrg_conv_El_to_Mec_Bosch/PTI_DriveEmot_Bosch/AWR 2 TX/Nm_to_percent ==
  Nm_Torque : Inport
  Reference_Torque : Inport  Port=2
  Constant : Constant  Value=100
  Divide1 : Product  Inputs=*/
  Product1 : Product  RndMeth=Zero
  Torque_Percentage : Outport
  wires:
  Nm_Torque/1 -> Divide1/1  "Nm_Torque"
  Product1/1 -> Torque_Percentage/1  "Torque_Percentage"
  Reference_Torque/1 -> Divide1/2  "Reference_Torque"
  Divide1/1 -> Product1/1
  Constant/1 -> Product1/2

== system Enrg_conv_El_to_Mec_Bosch/PTI_DriveEmot_Bosch/AWR 2 TX/Nm_to_percent1 ==
  Nm_Torque : Inport
  Reference_Torque : Inport  Port=2
  Constant : Constant  Value=100
  Divide1 : Product  Inputs=*/
  Product1 : Product  RndMeth=Zero
  Torque_Percentage : Outport
  wires:
  Constant/1 -> Product1/2
  Divide1/1 -> Product1/1
  Reference_Torque/1 -> Divide1/2  "Reference_Torque"
  Product1/1 -> Torque_Percentage/1  "Torque_Percentage"
  Nm_Torque/1 -> Divide1/1  "Nm_Torque"

== system Enrg_conv_El_to_Mec_Bosch/PTI_DriveEmot_Bosch/AWR 2 TX/Nm_to_percent2 ==
  Nm_Torque : Inport
  Reference_Torque : Inport  Port=2
  Constant : Constant  Value=100
  Divide1 : Product  Inputs=*/
  Product1 : Product  RndMeth=Zero
  Torque_Percentage : Outport
  wires:
  Nm_Torque/1 -> Divide1/1  "Nm_Torque"
  Product1/1 -> Torque_Percentage/1  "Torque_Percentage"
  Reference_Torque/1 -> Divide1/2  "Reference_Torque"
  Divide1/1 -> Product1/1
  Constant/1 -> Product1/2

== system Enrg_conv_El_to_Mec_Bosch/PTI_DriveEmot_Bosch/AWR 3 TX/Nm_to_percent ==
  Nm_Torque : Inport
  Reference_Torque : Inport  Port=2
  Constant : Constant  Value=100
  Divide1 : Product  Inputs=*/
  Product1 : Product  RndMeth=Zero
  Torque_Percentage : Outport
  wires:
  Constant/1 -> Product1/2
  Divide1/1 -> Product1/1
  Reference_Torque/1 -> Divide1/2  "Reference_Torque"
  Product1/1 -> Torque_Percentage/1  "Torque_Percentage"
  Nm_Torque/1 -> Divide1/1  "Nm_Torque"

== system Enrg_conv_El_to_Mec_Bosch/PTI_DriveEmot_Bosch/AWR 3 TX/Nm_to_percent1 ==
  Nm_Torque : Inport
  Reference_Torque : Inport  Port=2
  Constant : Constant  Value=100
  Divide1 : Product  Inputs=*/
  Product1 : Product  RndMeth=Zero
  Torque_Percentage : Outport
  wires:
  Nm_Torque/1 -> Divide1/1  "Nm_Torque"
  Product1/1 -> Torque_Percentage/1  "Torque_Percentage"
  Reference_Torque/1 -> Divide1/2  "Reference_Torque"
  Divide1/1 -> Product1/1
  Constant/1 -> Product1/2

== system Enrg_conv_El_to_Mec_Bosch/PTI_DriveEmot_Bosch/AWR 3 TX/Nm_to_percent2 ==
  Nm_Torque : Inport
  Reference_Torque : Inport  Port=2
  Constant : Constant  Value=100
  Divide1 : Product  Inputs=*/
  Product1 : Product  RndMeth=Zero
  Torque_Percentage : Outport
  wires:
  Constant/1 -> Product1/2
  Divide1/1 -> Product1/1
  Reference_Torque/1 -> Divide1/2  "Reference_Torque"
  Product1/1 -> Torque_Percentage/1  "Torque_Percentage"
  Nm_Torque/1 -> Divide1/1  "Nm_Torque"

== system Enrg_conv_El_to_Mec_Bosch/PTI_DriveEmot_Bosch/AWR 4 TX/Nm_to_percent ==
  Nm_Torque : Inport
  Reference_Torque : Inport  Port=2
  Constant : Constant  Value=100
  Divide1 : Product  Inputs=*/
  Product1 : Product  RndMeth=Zero
  Torque_Percentage : Outport
  wires:
  Constant/1 -> Product1/2
  Divide1/1 -> Product1/1
  Reference_Torque/1 -> Divide1/2  "Reference_Torque"
  Product1/1 -> Torque_Percentage/1  "Torque_Percentage"
  Nm_Torque/1 -> Divide1/1  "Nm_Torque"

== system Enrg_conv_El_to_Mec_Bosch/PTI_DriveEmot_Bosch/AWR 4 TX/Nm_to_percent1 ==
  Nm_Torque : Inport
  Reference_Torque : Inport  Port=2
  Constant : Constant  Value=100
  Divide1 : Product  Inputs=*/
  Product1 : Product  RndMeth=Zero
  Torque_Percentage : Outport
  wires:
  Nm_Torque/1 -> Divide1/1  "Nm_Torque"
  Product1/1 -> Torque_Percentage/1  "Torque_Percentage"
  Reference_Torque/1 -> Divide1/2  "Reference_Torque"
  Divide1/1 -> Product1/1
  Constant/1 -> Product1/2

== system Enrg_conv_El_to_Mec_Bosch/PTI_DriveEmot_Bosch/AWR 4 TX/Nm_to_percent2 ==
  Nm_Torque : Inport
  Reference_Torque : Inport  Port=2
  Constant : Constant  Value=100
  Divide1 : Product  Inputs=*/
  Product1 : Product  RndMeth=Zero
  Torque_Percentage : Outport
  wires:
  Constant/1 -> Product1/2
  Divide1/1 -> Product1/1
  Reference_Torque/1 -> Divide1/2  "Reference_Torque"
  Product1/1 -> Torque_Percentage/1  "Torque_Percentage"
  Nm_Torque/1 -> Divide1/1  "Nm_Torque"

== system Enrg_conv_El_to_Mec_Bosch/PTI_DriveEmot_Bosch/AWR1_4/ZeroWhenNotReady1 ==
  Bus Creator4 : BusCreator  Inputs=11
  zero_EMD1_ACT_DcLinkPower : Constant  Value=0
  zero_EMD1_ACT_DcLinkVoltage : Constant  Value=0
  zero_EMD1_ACT_DigitalInput1 : Constant  Value=0
  zero_EMD1_ACT_InverterState : Constant  Value=0
  zero_EMD1_ACT_MaxJunctionTemperature : Constant  Value=0
  zero_EMD1_ACT_MaximumAvailableTorque : Constant  Value=0
  zero_EMD1_ACT_MotorSpeed : Constant  Value=0
  zero_EMD1_ACT_MotorTemperature : Constant  Value=0
  zero_EMD1_ACT_MotorTorque : Constant  Value=0
  zero_EMD1_ACT_ReferenceTorqueLimited : Constant  Value=0
  zero_trqEmot1DesPhy : Constant  Value=0
  Out1 : Outport
  wires:
  Bus Creator4/1 -> Out1/1  "awr1B"
  zero_EMD1_ACT_DcLinkVoltage/1 -> Bus Creator4/1  "EMD1_ACT_DcLinkVoltage"
  zero_EMD1_ACT_DigitalInput1/1 -> Bus Creator4/2  "EMD_ACT_DigitalInput1"
  zero_EMD1_ACT_MaximumAvailableTorque/1 -> Bus Creator4/3  "EMD_ACT_MaximumAvailableTorque"
  zero_EMD1_ACT_DcLinkPower/1 -> Bus Creator4/4  "EMD_ACT_DcLinkPower"
  zero_EMD1_ACT_MotorSpeed/1 -> Bus Creator4/5  "EMD_ACT_MotorSpeed"
  zero_EMD1_ACT_MotorTorque/1 -> Bus Creator4/6  "EMD_ACT_MotorTorque"
  zero_EMD1_ACT_InverterState/1 -> Bus Creator4/7  "EMD_ACT_InverterState"
  zero_EMD1_ACT_ReferenceTorqueLimited/1 -> Bus Creator4/8  "EMD_ACT_ReferenceTorqueLimited"
  zero_trqEmot1DesPhy/1 -> Bus Creator4/9  "trqEmotDesPhy"
  zero_EMD1_ACT_MaxJunctionTemperature/1 -> Bus Creator4/10  "EMD_ACT_MaxJunctionTemperature"
  zero_EMD1_ACT_MotorTemperature/1 -> Bus Creator4/11  "EMD_ACT_MotorTemperature"

== system Enrg_conv_El_to_Mec_Bosch/PTI_DriveEmot_Bosch/AWR1_4/ZeroWhenNotReady2 ==
  Bus Creator4 : BusCreator  Inputs=11
  zero_EMD4_ACT_DcLinkPower : Constant  Value=0
  zero_EMD4_ACT_DcLinkVoltage : Constant  Value=0
  zero_EMD4_ACT_DigitalInput1 : Constant  Value=0
  zero_EMD4_ACT_InverterState : Constant  Value=0
  zero_EMD4_ACT_MaxJunctionTemperature : Constant  Value=0
  zero_EMD4_ACT_MaximumAvailableTorque : Constant  Value=0
  zero_EMD4_ACT_MotorSpeed : Constant  Value=0
  zero_EMD4_ACT_MotorTemperature : Constant  Value=0
  zero_EMD4_ACT_MotorTorque : Constant  Value=0
  zero_EMD4_ACT_ReferenceTorqueLimited : Constant  Value=0
  zero_trqEmot1DesPhy : Constant  Value=0
  Out1 : Outport
  wires:
  zero_EMD4_ACT_MotorTemperature/1 -> Bus Creator4/11  "EMD_ACT_MotorTemperature"
  zero_EMD4_ACT_MaxJunctionTemperature/1 -> Bus Creator4/10  "EMD_ACT_MaxJunctionTemperature"
  zero_trqEmot1DesPhy/1 -> Bus Creator4/9  "trqEmotDesPhy"
  zero_EMD4_ACT_ReferenceTorqueLimited/1 -> Bus Creator4/8  "EMD_ACT_ReferenceTorqueLimited"
  zero_EMD4_ACT_InverterState/1 -> Bus Creator4/7  "EMD_ACT_InverterState"
  zero_EMD4_ACT_MotorTorque/1 -> Bus Creator4/6  "EMD_ACT_MotorTorque"
  zero_EMD4_ACT_MotorSpeed/1 -> Bus Creator4/5  "EMD_ACT_MotorSpeed"
  zero_EMD4_ACT_DcLinkPower/1 -> Bus Creator4/4  "EMD_ACT_DcLinkPower"
  zero_EMD4_ACT_MaximumAvailableTorque/1 -> Bus Creator4/3  "EMD_ACT_MaximumAvailableTorque"
  zero_EMD4_ACT_DigitalInput1/1 -> Bus Creator4/2  "EMD_ACT_DigitalInput1"
  zero_EMD4_ACT_DcLinkVoltage/1 -> Bus Creator4/1  "EMD4_ACT_DcLinkVoltage"
  Bus Creator4/1 -> Out1/1  "awr1B"

== system Enrg_conv_El_to_Mec_Bosch/PTI_DriveEmot_Bosch/AWR2_3/ZeroWhenNotReady1 ==
  Bus Creator4 : BusCreator  Inputs=11
  zero_EMD1_ACT_DcLinkPower : Constant  Value=0
  zero_EMD1_ACT_DigitalInput1 : Constant  Value=0
  zero_EMD1_ACT_InverterState : Constant  Value=0
  zero_EMD1_ACT_MaxJunctionTemperature : Constant  Value=0
  zero_EMD1_ACT_MaximumAvailableTorque : Constant  Value=0
  zero_EMD1_ACT_MotorSpeed : Constant  Value=0
  zero_EMD1_ACT_MotorTemperature : Constant  Value=0
  zero_EMD1_ACT_MotorTorque : Constant  Value=0
  zero_EMD1_ACT_ReferenceTorqueLimited : Constant  Value=0
  zero_EMD2_ACT_DcLinkVoltage : Constant  Value=0
  zero_trqEmot1DesPhy : Constant  Value=0
  Out1 : Outport
  wires:
  zero_EMD1_ACT_MotorTemperature/1 -> Bus Creator4/11  "EMD_ACT_MotorTemperature"
  zero_EMD1_ACT_MaxJunctionTemperature/1 -> Bus Creator4/10  "EMD_ACT_MaxJunctionTemperature"
  zero_trqEmot1DesPhy/1 -> Bus Creator4/9  "trqEmotDesPhy"
  zero_EMD1_ACT_ReferenceTorqueLimited/1 -> Bus Creator4/8  "EMD_ACT_ReferenceTorqueLimited"
  zero_EMD1_ACT_InverterState/1 -> Bus Creator4/7  "EMD_ACT_InverterState"
  zero_EMD1_ACT_MotorTorque/1 -> Bus Creator4/6  "EMD_ACT_MotorTorque"
  zero_EMD1_ACT_MotorSpeed/1 -> Bus Creator4/5  "EMD_ACT_MotorSpeed"
  zero_EMD1_ACT_DcLinkPower/1 -> Bus Creator4/4  "EMD_ACT_DcLinkPower"
  zero_EMD1_ACT_MaximumAvailableTorque/1 -> Bus Creator4/3  "EMD_ACT_MaximumAvailableTorque"
  zero_EMD1_ACT_DigitalInput1/1 -> Bus Creator4/2  "EMD_ACT_DigitalInput1"
  zero_EMD2_ACT_DcLinkVoltage/1 -> Bus Creator4/1  "EMD2_ACT_DcLinkVoltage"
  Bus Creator4/1 -> Out1/1  "awr2B"

== system Enrg_conv_El_to_Mec_Bosch/PTI_DriveEmot_Bosch/AWR2_3/ZeroWhenNotReady2 ==
  Bus Creator4 : BusCreator  Inputs=11
  zero_EMD3_ACT_DcLinkVoltage : Constant  Value=0
  zero_EMD4_ACT_DcLinkPower : Constant  Value=0
  zero_EMD4_ACT_DigitalInput1 : Constant  Value=0
  zero_EMD4_ACT_InverterState : Constant  Value=0
  zero_EMD4_ACT_MaxJunctionTemperature : Constant  Value=0
  zero_EMD4_ACT_MaximumAvailableTorque : Constant  Value=0
  zero_EMD4_ACT_MotorSpeed : Constant  Value=0
  zero_EMD4_ACT_MotorTemperature : Constant  Value=0
  zero_EMD4_ACT_MotorTorque : Constant  Value=0
  zero_EMD4_ACT_ReferenceTorqueLimited : Constant  Value=0
  zero_trqEmot1DesPhy : Constant  Value=0
  Out1 : Outport
  wires:
  Bus Creator4/1 -> Out1/1  "awr3B"
  zero_EMD3_ACT_DcLinkVoltage/1 -> Bus Creator4/1  "EMD3_ACT_DcLinkVoltage"
  zero_EMD4_ACT_DigitalInput1/1 -> Bus Creator4/2  "EMD_ACT_DigitalInput1"
  zero_EMD4_ACT_MaximumAvailableTorque/1 -> Bus Creator4/3  "EMD_ACT_MaximumAvailableTorque"
  zero_EMD4_ACT_DcLinkPower/1 -> Bus Creator4/4  "EMD_ACT_DcLinkPower"
  zero_EMD4_ACT_MotorSpeed/1 -> Bus Creator4/5  "EMD_ACT_MotorSpeed"
  zero_EMD4_ACT_MotorTorque/1 -> Bus Creator4/6  "EMD_ACT_MotorTorque"
  zero_EMD4_ACT_InverterState/1 -> Bus Creator4/7  "EMD_ACT_InverterState"
  zero_EMD4_ACT_ReferenceTorqueLimited/1 -> Bus Creator4/8  "EMD_ACT_ReferenceTorqueLimited"
  zero_trqEmot1DesPhy/1 -> Bus Creator4/9  "trqEmotDesPhy"
  zero_EMD4_ACT_MaxJunctionTemperature/1 -> Bus Creator4/10  "EMD_ACT_MaxJunctionTemperature"
  zero_EMD4_ACT_MotorTemperature/1 -> Bus Creator4/11  "EMD_ACT_MotorTemperature"

== system Enrg_conv_El_to_Mec_Bosch/PTI_DriveEmot_Bosch/EMD1_CMD_Command/Compare To Constant ==
  u : Inport
  Compare : RelationalOperator  Operator===  OutDataTypeStr=boolean  InputSameDT=on
  Constant : Constant  DisableCoverage=on  Value=const  OutDataTypeStr=Inherit: Inherit via back propagation
  y : Outport
  wires:
  Compare/1 -> y/1
  Constant/1 -> Compare/2
  u/1 -> Compare/1

== system Enrg_conv_El_to_Mec_Bosch/PTI_DriveEmot_Bosch/EMD1_CMD_Command/Compare To Constant1 ==
  u : Inport
  Compare : RelationalOperator  Operator===  OutDataTypeStr=boolean  InputSameDT=on
  Constant : Constant  DisableCoverage=on  Value=const  OutDataTypeStr=Inherit: Inherit via back propagation
  y : Outport
  wires:
  Compare/1 -> y/1
  Constant/1 -> Compare/2
  u/1 -> Compare/1

== system Enrg_conv_El_to_Mec_Bosch/PTI_DriveEmot_Bosch/EMD1_CMD_Command1/Compare To Constant ==
  u : Inport
  Compare : RelationalOperator  Operator===  OutDataTypeStr=boolean  InputSameDT=on
  Constant : Constant  DisableCoverage=on  Value=const  OutDataTypeStr=Inherit: Inherit via back propagation
  y : Outport
  wires:
  Compare/1 -> y/1
  Constant/1 -> Compare/2
  u/1 -> Compare/1

== system Enrg_conv_El_to_Mec_Bosch/PTI_DriveEmot_Bosch/EMD1_CMD_Command1/Compare To Constant1 ==
  u : Inport
  Compare : RelationalOperator  Operator===  OutDataTypeStr=boolean  InputSameDT=on
  Constant : Constant  DisableCoverage=on  Value=const  OutDataTypeStr=Inherit: Inherit via back propagation
  y : Outport
  wires:
  Compare/1 -> y/1
  Constant/1 -> Compare/2
  u/1 -> Compare/1

== system Enrg_conv_El_to_Mec_Bosch/PTI_DriveEmot_Bosch/EMD1_CMD_Command2/Compare To Constant ==
  u : Inport
  Compare : RelationalOperator  Operator===  OutDataTypeStr=boolean  InputSameDT=on
  Constant : Constant  DisableCoverage=on  Value=const  OutDataTypeStr=Inherit: Inherit via back propagation
  y : Outport
  wires:
  Compare/1 -> y/1
  Constant/1 -> Compare/2
  u/1 -> Compare/1

== system Enrg_conv_El_to_Mec_Bosch/PTI_DriveEmot_Bosch/EMD1_CMD_Command2/Compare To Constant1 ==
  u : Inport
  Compare : RelationalOperator  Operator===  OutDataTypeStr=boolean  InputSameDT=on
  Constant : Constant  DisableCoverage=on  Value=const  OutDataTypeStr=Inherit: Inherit via back propagation
  y : Outport
  wires:
  Compare/1 -> y/1
  Constant/1 -> Compare/2
  u/1 -> Compare/1

== system Enrg_conv_El_to_Mec_Bosch/PTI_DriveEmot_Bosch/EMD1_CMD_Command3/Compare To Constant ==
  u : Inport
  Compare : RelationalOperator  Operator===  OutDataTypeStr=boolean  InputSameDT=on
  Constant : Constant  DisableCoverage=on  Value=const  OutDataTypeStr=Inherit: Inherit via back propagation
  y : Outport
  wires:
  Compare/1 -> y/1
  Constant/1 -> Compare/2
  u/1 -> Compare/1

== system Enrg_conv_El_to_Mec_Bosch/PTI_DriveEmot_Bosch/EMD1_CMD_Command3/Compare To Constant1 ==
  u : Inport
  Compare : RelationalOperator  Operator===  OutDataTypeStr=boolean  InputSameDT=on
  Constant : Constant  DisableCoverage=on  Value=const  OutDataTypeStr=Inherit: Inherit via back propagation
  y : Outport
  wires:
  Compare/1 -> y/1
  Constant/1 -> Compare/2
  u/1 -> Compare/1

== system Enrg_conv_El_to_Mec_Bosch/PTI_DriveEmot_Bosch_10ms/AWR1_4/ZeroWhenNotReady1 ==
  Bus Creator4 : BusCreator  Inputs=11
  zero_EMD1_ACT_DcLinkPower : Constant  Value=0
  zero_EMD1_ACT_DcLinkVoltage : Constant  Value=0
  zero_EMD1_ACT_DigitalInput1 : Constant  Value=0
  zero_EMD1_ACT_InverterState : Constant  Value=0
  zero_EMD1_ACT_MaxJunctionTemperature : Constant  Value=0
  zero_EMD1_ACT_MaximumAvailableTorque : Constant  Value=0
  zero_EMD1_ACT_MotorSpeed : Constant  Value=0
  zero_EMD1_ACT_MotorTemperature : Constant  Value=0
  zero_EMD1_ACT_MotorTorque : Constant  Value=0
  zero_EMD1_ACT_ReferenceTorqueLimited : Constant  Value=0
  zero_trqEmot1DesPhy : Constant  Value=0
  Out1 : Outport
  wires:
  zero_EMD1_ACT_MotorTemperature/1 -> Bus Creator4/11  "EMD_ACT_MotorTemperature"
  zero_EMD1_ACT_MaxJunctionTemperature/1 -> Bus Creator4/10  "EMD_ACT_MaxJunctionTemperature"
  zero_trqEmot1DesPhy/1 -> Bus Creator4/9  "trqEmotDesPhy"
  zero_EMD1_ACT_ReferenceTorqueLimited/1 -> Bus Creator4/8  "EMD_ACT_ReferenceTorqueLimited"
  zero_EMD1_ACT_InverterState/1 -> Bus Creator4/7  "EMD_ACT_InverterState"
  zero_EMD1_ACT_MotorTorque/1 -> Bus Creator4/6  "EMD_ACT_MotorTorque"
  zero_EMD1_ACT_MotorSpeed/1 -> Bus Creator4/5  "EMD_ACT_MotorSpeed"
  zero_EMD1_ACT_DcLinkPower/1 -> Bus Creator4/4  "EMD_ACT_DcLinkPower"
  zero_EMD1_ACT_MaximumAvailableTorque/1 -> Bus Creator4/3  "EMD_ACT_MaximumAvailableTorque"
  zero_EMD1_ACT_DigitalInput1/1 -> Bus Creator4/2  "EMD_ACT_DigitalInput1"
  zero_EMD1_ACT_DcLinkVoltage/1 -> Bus Creator4/1  "EMD1_ACT_DcLinkVoltage"
  Bus Creator4/1 -> Out1/1  "awr1B"

== system Enrg_conv_El_to_Mec_Bosch/PTI_DriveEmot_Bosch_10ms/AWR1_4/ZeroWhenNotReady2 ==
  Bus Creator4 : BusCreator  Inputs=11
  zero_EMD4_ACT_DcLinkPower : Constant  Value=0
  zero_EMD4_ACT_DcLinkVoltage : Constant  Value=0
  zero_EMD4_ACT_DigitalInput1 : Constant  Value=0
  zero_EMD4_ACT_InverterState : Constant  Value=0
  zero_EMD4_ACT_MaxJunctionTemperature : Constant  Value=0
  zero_EMD4_ACT_MaximumAvailableTorque : Constant  Value=0
  zero_EMD4_ACT_MotorSpeed : Constant  Value=0
  zero_EMD4_ACT_MotorTemperature : Constant  Value=0
  zero_EMD4_ACT_MotorTorque : Constant  Value=0
  zero_EMD4_ACT_ReferenceTorqueLimited : Constant  Value=0
  zero_trqEmot1DesPhy : Constant  Value=0
  Out1 : Outport
  wires:
  Bus Creator4/1 -> Out1/1  "awr1B"
  zero_EMD4_ACT_DcLinkVoltage/1 -> Bus Creator4/1  "EMD4_ACT_DcLinkVoltage"
  zero_EMD4_ACT_DigitalInput1/1 -> Bus Creator4/2  "EMD_ACT_DigitalInput1"
  zero_EMD4_ACT_MaximumAvailableTorque/1 -> Bus Creator4/3  "EMD_ACT_MaximumAvailableTorque"
  zero_EMD4_ACT_DcLinkPower/1 -> Bus Creator4/4  "EMD_ACT_DcLinkPower"
  zero_EMD4_ACT_MotorSpeed/1 -> Bus Creator4/5  "EMD_ACT_MotorSpeed"
  zero_EMD4_ACT_MotorTorque/1 -> Bus Creator4/6  "EMD_ACT_MotorTorque"
  zero_EMD4_ACT_InverterState/1 -> Bus Creator4/7  "EMD_ACT_InverterState"
  zero_EMD4_ACT_ReferenceTorqueLimited/1 -> Bus Creator4/8  "EMD_ACT_ReferenceTorqueLimited"
  zero_trqEmot1DesPhy/1 -> Bus Creator4/9  "trqEmotDesPhy"
  zero_EMD4_ACT_MaxJunctionTemperature/1 -> Bus Creator4/10  "EMD_ACT_MaxJunctionTemperature"
  zero_EMD4_ACT_MotorTemperature/1 -> Bus Creator4/11  "EMD_ACT_MotorTemperature"

== system Enrg_conv_El_to_Mec_Bosch/PTI_DriveEmot_Bosch_10ms/AWR2_3/ZeroWhenNotReady1 ==
  Bus Creator4 : BusCreator  Inputs=11
  zero_EMD1_ACT_DcLinkPower : Constant  Value=0
  zero_EMD1_ACT_DigitalInput1 : Constant  Value=0
  zero_EMD1_ACT_InverterState : Constant  Value=0
  zero_EMD1_ACT_MaxJunctionTemperature : Constant  Value=0
  zero_EMD1_ACT_MaximumAvailableTorque : Constant  Value=0
  zero_EMD1_ACT_MotorSpeed : Constant  Value=0
  zero_EMD1_ACT_MotorTemperature : Constant  Value=0
  zero_EMD1_ACT_MotorTorque : Constant  Value=0
  zero_EMD1_ACT_ReferenceTorqueLimited : Constant  Value=0
  zero_EMD2_ACT_DcLinkVoltage : Constant  Value=0
  zero_trqEmot1DesPhy : Constant  Value=0
  Out1 : Outport
  wires:
  Bus Creator4/1 -> Out1/1  "awr2B"
  zero_EMD2_ACT_DcLinkVoltage/1 -> Bus Creator4/1  "EMD2_ACT_DcLinkVoltage"
  zero_EMD1_ACT_DigitalInput1/1 -> Bus Creator4/2  "EMD_ACT_DigitalInput1"
  zero_EMD1_ACT_MaximumAvailableTorque/1 -> Bus Creator4/3  "EMD_ACT_MaximumAvailableTorque"
  zero_EMD1_ACT_DcLinkPower/1 -> Bus Creator4/4  "EMD_ACT_DcLinkPower"
  zero_EMD1_ACT_MotorSpeed/1 -> Bus Creator4/5  "EMD_ACT_MotorSpeed"
  zero_EMD1_ACT_MotorTorque/1 -> Bus Creator4/6  "EMD_ACT_MotorTorque"
  zero_EMD1_ACT_InverterState/1 -> Bus Creator4/7  "EMD_ACT_InverterState"
  zero_EMD1_ACT_ReferenceTorqueLimited/1 -> Bus Creator4/8  "EMD_ACT_ReferenceTorqueLimited"
  zero_trqEmot1DesPhy/1 -> Bus Creator4/9  "trqEmotDesPhy"
  zero_EMD1_ACT_MaxJunctionTemperature/1 -> Bus Creator4/10  "EMD_ACT_MaxJunctionTemperature"
  zero_EMD1_ACT_MotorTemperature/1 -> Bus Creator4/11  "EMD_ACT_MotorTemperature"
